simulink model "Problem2_3_2"  (R2018a)
settings: Solver=VariableStepAuto  StartTime=0.0  StopTime=100  RelTol=1e-3
settings Model: Creator=NIMA  LastModifiedBy=NIMA

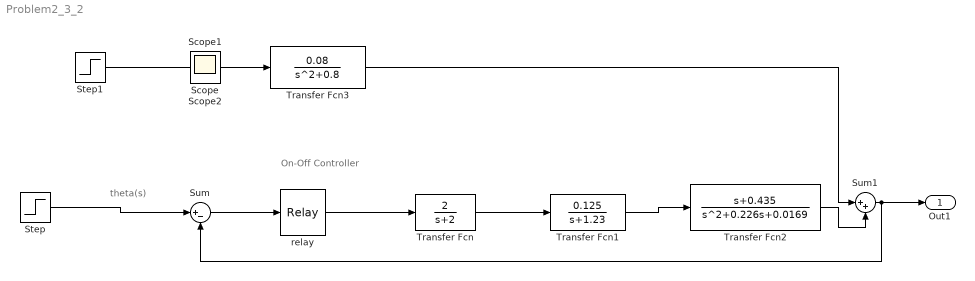
== system Problem2_3_2 ==
  note: On-Off
      | Controller
  note: theta(s)
  Step : Step  SampleTime=0
  Step1 : Step  Time=40  SampleTime=0
  Sum : Sum  Inputs=|+-
  Sum1 : Sum  Inputs=|++
  Transfer Fcn : TransferFcn  Numerator=[2]  Denominator=[1 2]
  Transfer Fcn1 : TransferFcn  Numerator=[0.125]  Denominator=[1 1.23]
  Transfer Fcn2 : TransferFcn  Numerator=[1 0.435]  Denominator=[1 0.226 0.0169]
  Transfer Fcn3 : TransferFcn  Numerator=[0.08]  Denominator=[1 0 0.8]
  relay : Relay  OnSwitchValue=0.001  OffSwitchValue=-0.001  OnOutputValue=1.15  OffOutputValue=-1.15
  Out1 : Outport
  Scope : Scope
  Scope1 : Scope
  Scope2 : Scope
  wires:
  Step1/1 -> Transfer Fcn3/1
  Transfer Fcn/1 -> Transfer Fcn1/1
  relay/1 -> Transfer Fcn/1
  Sum/1 -> relay/1
  Step/1 -> Sum/1
  Transfer Fcn1/1 -> Transfer Fcn2/1
  Transfer Fcn2/1 -> Sum1/2
  Transfer Fcn3/1 -> Sum1/1
  Sum1/1 -> Out1/1, Sum/2
